simulink model "MatMul_int32"  (R2025a)
settings: Solver=VariableStepAuto  StartTime=0.0  StopTime=62  RelTol=1e-3
undefined symbols (not defined in the file): S, vsva2197, xcvc1902
libraries: aieBasic x1, vmcUtilities x1, aieUtilities x1
settings Model: Creator=niteshp  LastModifiedBy=sdegala
settings SolverCC: AlgebraicLoopSolver=TrustRegion
settings DebuggingCC: UnconnectedInputMsg=warning  UnconnectedOutputMsg=warning  UnconnectedLineMsg=warning
settings ModelReferenceCC: EnableRefExpFcnMdlSchedulingChecks=on
settings RTWCC: GPUComputeCapability=3.5  DLArmComputeVersion=19.05

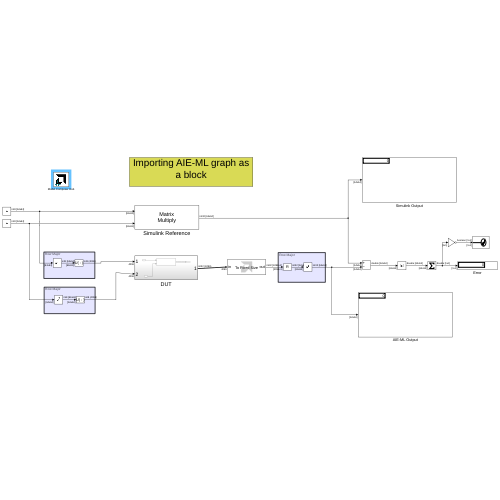
[thumbnail: Simulink's stored preview of the top-level diagram]
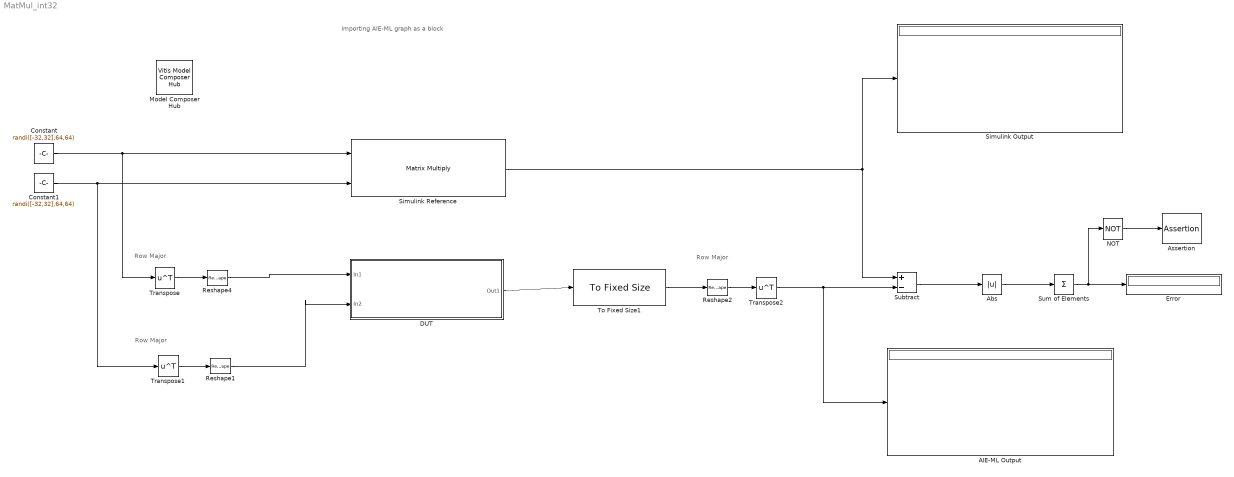
== system MatMul_int32 ==
  note: Row Major
  note: Row Major
  note: Row Major
  note: Importing AIE-ML graph as a block
  AIE-ML Output : Display
  Abs : Abs  SaturateOnIntegerOverflow=off
  Assertion : Assertion
  Constant : Constant  Value=randi([-32,32],64,64)  VectorParams1D=off  OutDataTypeStr=int8  SampleTime=1
  Constant1 : Constant  Value=randi([-32,32],64,64)  VectorParams1D=off  OutDataTypeStr=int8  SampleTime=1
  DUT : Subsystem
  Error : Display
  Model Composer Hub : vmcUtilities/Vitis Model Composer Hub  Tag=genX  Description=Performs multiplication  CodeGeneration=off  SubsystemName=DUT  BlockHierPath=MatMul_int32/DUT  SubsystemType=AIENode  AIEArrayConfig=Use entire AIE array  StartColumn=1  NumberOfColumns=1  TargetDirectory=./code  exportDesign=on  analyzeDesign=off  validateDesignOnHw=off  ExportType=AI Engines  IpVendor=xilinx.com  IpLibrary=hls  IpVersion=1.0  IpHWLanguage=Verilog  AieCompilerOptions={}  AieSimulatorOptions={}  CreateTestbench=on  TestbenchStackSize=10  RunRtlSim=off  RunCSim=off  RunAieSim=on  AieSimTimeout=50000  RunAieSimProfiling=off  LaunchVitisAnalyzer=off  PlotOutput=off  RunX86Sim=on  X86SimTimeout=10  GenHwImage=off  GenLibadfXo=off  GenHwValidationCode=off  PlatformType=Specify Platform  Platform=/proj/xbuilds/SWIP/9999.0_0818_1732/installs/lin64/2025.2/Vitis/base_platforms/xilinx_vck190_base_202520_1/xilinx_vck190_base_202520_1.xpfm  HwSystemType=Baremetal  HwValidationTarget=hw  ProjDevice=Versal VCK190 Evaluation Platform (xcvc1902-vsva2197-2MP-e-S)  ProjDevicePart=xcvc1902-vsva2197-2MP-e-S  AIEType=AIE  SamplePeriod=-1  ClockFrequency=200  DataPathParallelism=1  xilinxfamily=versalaicore  part=xcvc1902  speed=-2MP-e-S  package=vsva2197  directory=./netlist  testbench=off  incr_netlist=off  synthesis_tool=Vivado  clock_wrapper=Clock Enables  dbl_ovrd=According to Block Masks  dcm_input_clock_period=10  sysclk_period=10  simulink_period=1  eval_field=0  IPInfoJsonString="{\"DUTSubsystemName\":\"DUT\",\"AIESubsystem\":{\"SubsystemName\":\"DUT\",\"TargetDirectory\":\"./code\",\"AIEArrayConfig\":\"Use entire AIE array\",\"StartColumn\":\"0\",\"NumberOfColumns\":\"1\"},\"SubsystemTag\":\"AIENode\"}"  LogFileName=/proj/xhdhdstaff5/sdegala/Head1/HEAD/VMC_2025_2_July/Examples/AIENGINE/Importing_AIE_blocks/AIE_ML_Graph_Import/code/model_composer.log  NThreads=4  IPConfigFile=/tmp/vmctmp-6835010160091439353/MatMul_int32_ipconfig.json
  NOT : Logic  Operator=NOT  IconShape=distinctive  AllPortsSameDT=off  OutDataTypeStr=boolean
  Reshape1 : Reshape  OutputDimensions=[16,16]
  Reshape2 : Reshape  OutputDimensionality=Customize  OutputDimensions=[64,64]
  Reshape4 : Reshape  OutputDimensions=[16,16]
  Simulink Output : Display
  Simulink Reference : Product  Multiplication=Matrix(*)  OutDataTypeStr=int32
  Subtract : Sum  Inputs=+-  OutDataTypeStr=double
  Sum of Elements : Sum  Inputs=+
  To Fixed Size1 : aieUtilities/To Fixed Size  Mode=Stop simulation when input variable-size signal is not full  OutputSize=Inherit: Same as input  CopyMethod=Buffer samples to form output  HasStatusOutput=off
  Transpose : Math  Operator=transpose
  Transpose1 : Math  Operator=transpose
  Transpose2 : Math  Operator=transpose
  wires:
  Constant/1 -> Transpose/1, Simulink Reference/1
  To Fixed Size1/1 -> Reshape2/1
  Simulink Reference/1 -> Subtract/1, Simulink Output/1
  Subtract/1 -> Abs/1
  Abs/1 -> Sum of Elements/1
  Reshape2/1 -> Transpose2/1
  Constant1/1 -> Transpose1/1, Simulink Reference/2
  DUT/1(Out1) -> To Fixed Size1/1
  Reshape4/1 -> DUT/1(In1)
  Reshape1/1 -> DUT/2(In2)
  Sum of Elements/1 -> NOT/1, Error/1
  NOT/1 -> Assertion/1
  Transpose/1 -> Reshape4/1
  Transpose1/1 -> Reshape1/1
  Transpose2/1 -> AIE-ML Output/1, Subtract/2

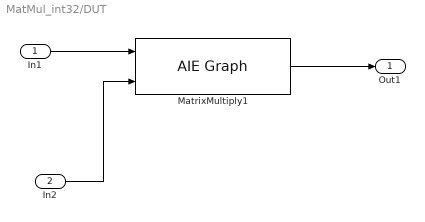
== system MatMul_int32/DUT ==
  In1 : Inport
  In2 : Inport  Port=2
  MatrixMultiply1 : aieBasic/AIE Graph  PortAttributesTable={ 'Input', 'inA', 'dma', 'int8', '64*64', 'sync', ''; 'Input', 'inB', 'dma', 'int8', '64*64', 'sync', ''; 'Output', 'outC', 'dma', 'int32', '64*64', 'sync', '' }  PortAttributesEnablement={'off', 'on', 'off', 'off', 'on', 'off', 'off';'off', 'on', 'off', 'off', 'on', 'off', 'off';'off', 'on', 'off', 'off', 'on', 'off', 'off'}  SampleTime=-1  ClassDeclTypeOptions=C[1 1]@t97@template < typename ITYPE, typename OTYPE, int SHIFT_RESULT, int ARRAY_COL > class MatrixMultiply  ClassDecl=template < typename ITYPE, typename OTYPE, int SHIFT_RESULT, int ARRAY_COL > class MatrixMultiply  ClassTemplateParams={'ITYPE', 'typename', 'int8';'OTYPE', 'typename', 'int32';'SHIFT_RESULT', 'int', '0';'ARRAY_COL', 'int', '10'}  ClassTemplateParamsEnables={'off', 'off', 'on';'off', 'off', 'on';'off', 'off', 'on';'off', 'off', 'on'}  ClassCtorDeclTypeOptions=C[1 1]@t7@<empty>  ClassCtorDecl=<empty>  ClassCtorParams={}  GraphAllAttrs=|  PortArgDecls={'in dma int8 in1'; 'in dma int8 in2'; 'out dma int32 out1'}  PortGraphPortNames={'inA'; 'inB'; 'outC'}  HierGraphPortNames={'inA'; 'inB'; 'outC'}  PortTypes={'dma'; 'dma'; 'dma'}  PortDataTypes={'int8'; 'int8'; 'int32'}  PortSizes={4.096000000000000000e+03; 4.096000000000000000e+03; 4.096000000000000000e+03}  PortSynchronicities={'sync'; 'sync'; 'sync'}  PortSignalSizes={0.000000000000000000e+00; 0.000000000000000000e+00; 0.000000000000000000e+00}  SimLibPath=''  ClassIndex=1  ClassCtorIndex=0  ClassTabVisible=on  FunctionTabVisible=on  DelayDrawLabels=off  GraphFileSelect=Header file (*.h)  GraphHeaderFile=src/MultGraph.h  GraphClassName=MatrixMultiply  GraphName=MatrixMultiply<signed char, int, 0, 10>  GraphHeaderFiles={'src/MultGraph.h'}  GraphSourceFile=./model_composer_work/xmc_aie_lib/3ddf452b/mygraph.cpp  GraphSearchPaths={}  GraphPreProcOptions={}  blockJsonConstraints=[]
      | s[12;12;9;9;19;14;21;23;21;23;24;21;15;17;12;24;26;26;26;27;28;9;21;23;23;23;24;25;14;19;19;29]@FunctionNameDeclFileNamePortNamesPortTypesPortSerializedTypesPortDirectionsPortWindowSizeEnablesPortWindowMarginEnablesPortBufferSizeEnablesPortBufferMarginEnablesPortSynchronicityEnablesPortSignalSizeEnablesPortBufferSizesPortBufferMarginsFunctionDeclFunctionTemplateSpecKindFunctionTemplateParamNamesFunctionTemplateParamKindsFunctionTemplateParamTypesFunctionTemplateParamValuesFunctionTemplateParamEnablesClassDeclClassTemplateSpecKindClassTemplateParamNamesClassTemplateParamKindsClassTemplateParamTypesClassTemplateParamValuesClassTemplateParamEnablesClassCtorDeclsClassCtorParamNamesClassCtorParamTypesClassCtorParamSerializedTypes[1 1]@C[32 1]@nt21@../../src/MultGraph.hC[3 1]@t3@inAt3@inBt4@outCC[3 1]@t31@adf::port< adf::direction::in >t31@adf::port< adf::direction::in >t32@adf::port< adf::direction::out >C[3 1]@t39@{Tadf::port{1{t{Sadf::direction::in}}}}t39@{Tadf::port{1{t{Sadf::direction::in}}}}t40@{Tadf::port{1{t{Sadf::direction::out}}}}C[3 1]@t5@inputt5@inputt5@inputC[3 1]@l0@l0@l0@C[3 1]@l0@l0@l0@C[3 1]@l0@l0@l0@C[3 1]@l0@l0@l0@C[3 1]@l1@l1@l1@C[3 1]@l0@l0@l0@C[3 1]@nnnC[3 1]@nnnt213@template < typename ITYPE, typename OTYPE, int SHIFT_RESULT, int ARRAY_COL > 
      | void MatrixMultiply::
      | (adf::port< adf::direction::in > inA, adf::port< adf::direction::in > inB, adf::port< adf::direction::out > outC)ne[0 1]@e[0 1]@e[0 1]@e[0 1]@e[0 1]@t98@template < typename ITYPE, typename OTYPE, int SHIFT_RESULT, int ARRAY_COL > class MatrixMultiply;t8@implicitC[4 1]@t5@ITYPEt5@OTYPEt12@SHIFT_RESULTt9@ARRAY_COLC[4 1]@t4@typet4@typet7@nontypet7@nontypeC[4 1]@t8@typenamet8@typenamet3@intt3@intC[4 1]@nnnnC[4 1]@l1@l1@l1@l1@e[0 1]@e[0 1]@e[0 1]@e[0 1]@
  Out1 : Outport
  wires:
  In1/1 -> MatrixMultiply1/1
  In2/1 -> MatrixMultiply1/2
  MatrixMultiply1/1 -> Out1/1
